simulink model "Control_movimiento_PID"  (R2021a)
settings: Solver=VariableStepAuto  StartTime=0.0  StopTime=10.0  RelTol=1e-3
undefined symbols (not defined in the file): ba, ksa, ksia
settings Model: Creator=fhlla  LastModifiedBy=fhlla

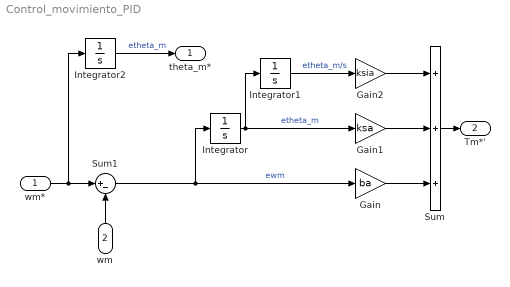
== system Control_movimiento_PID ==
  wm* : Inport
  wm : Inport  Port=2
  Gain : Gain  Gain=ba
  Gain1 : Gain  Gain=ksa
  Gain2 : Gain  Gain=ksia
  Integrator : Integrator
  Integrator1 : Integrator
  Integrator2 : Integrator
  Sum : Sum  Inputs=+++
  Sum1 : Sum  Inputs=|+-
  theta_m* : Outport
  Tm*' : Outport  Port=2
  wires:
  Gain2/1 -> Sum/1
  Integrator2/1 -> theta_m*/1  "etheta_m"
  Integrator1/1 -> Gain2/1  "etheta_m/s"
  Gain1/1 -> Sum/2
  Integrator/1 -> Integrator1/1, Gain1/1  "etheta_m"
  Gain/1 -> Sum/3
  wm/1 -> Sum1/2
  Sum1/1 -> Integrator/1, Gain/1  "ewm"
  wm*/1 -> Integrator2/1, Sum1/1
  Sum/1 -> Tm*'/1
